simulink model "closedloopsystem"  (R2018a)
settings: Solver=VariableStepAuto  StartTime=0.0  StopTime=25  RelTol=1e-3
values from neighbouring files (symbols this model uses):
  b = 0.1    [DC_Motormfile.m]
  JM = 0.4    [DC_Motormfile.m]
  KE = 0.12    [DC_Motormfile.m]    (also in pid.m)
  KT = 0.25    [DC_Motormfile.m]    (also in pid.m)
  L = 493*10^-9    (= 4.93e-07)    [DC_Motormfile.m]    (also in pid.m)
  R = 5.3*10^-3    (= 0.0053)    [DC_Motormfile.m]    (also in pid.m)
  Scaling_Velocity = Sc/(Cw)*Rg*KE    (= 4.865)    [pid.m]
libraries: simulink x1
settings Model: Creator=MAFAZ  LastModifiedBy=MAFAZ

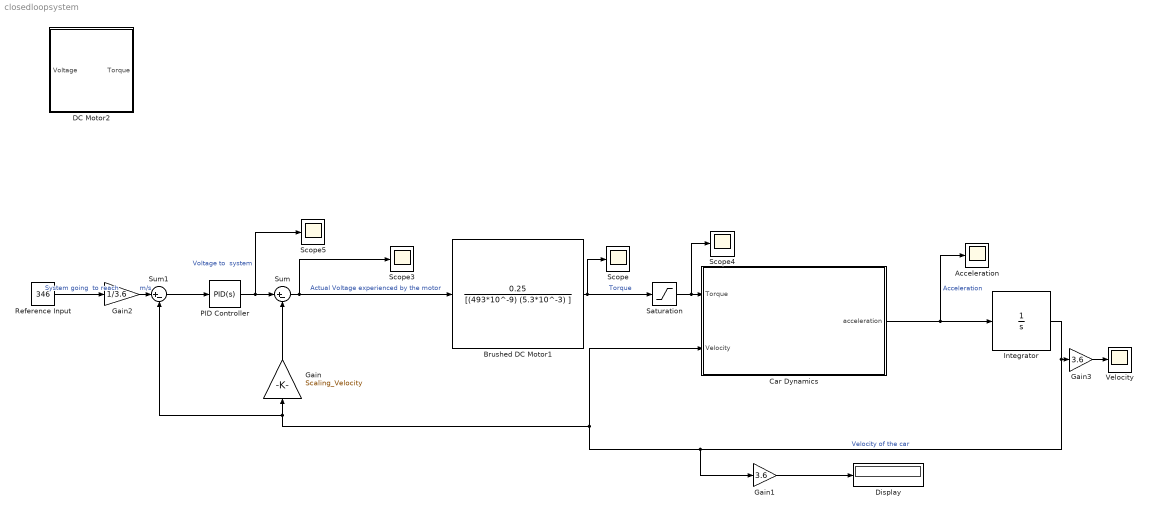
== system closedloopsystem ==
  Acceleration : Scope
  Brushed DC Motor1 : TransferFcn  Numerator=[0.25]  Denominator=[(493*10^-9) (5.3*10^-3) ]
  Car Dynamics : MATLAB Function  TreatAsAtomicUnit=on
  DC Motor2 : Subsystem
  Display : Display
  Gain : Gain  Gain=Scaling_Velocity
  Gain1 : Gain  Gain=3.6
  Gain2 : Gain  Gain=1/3.6
  Gain3 : Gain  Gain=3.6
  Integrator : Integrator
  PID Controller : simulink/Continuous/PID Controller  Controller=PID  TimeDomain=Continuous-time  SampleTime=-1  IntegratorMethod=Forward Euler  FilterMethod=Forward Euler  Form=Parallel  UseFilter=on  ControllerParametersSource=internal  P=1000000  I=0  D=0  N=100  InitialConditionSource=internal  InitialConditionForIntegrator=0  InitialConditionForFilter=0  ExternalReset=none  LimitOutput=on  UpperSaturationLimit=346  LowerSaturationLimit=0  LinearizeAsGain=on  AntiWindupMode=none  Kb=1  TrackingMode=off  Kt=1  PParamMin=[]  PParamMax=[]  IParamMin=[]  IParamMax=[]  DParamMin=[]  DParamMax=[]  NParamMin=[]  NParamMax=[]  KbParamMin=[]  KbParamMax=[]  KtParamMin=[]  KtParamMax=[]  POutMin=[]  POutMax=[]  IOutMin=[]  IOutMax=[]  DOutMin=[]  DOutMax=[]  NOutMin=[]  NOutMax=[]  KbOutMin=[]  KbOutMax=[]  KtOutMin=[]  KtOutMax=[]  IntegratorOutMin=[]  IntegratorOutMax=[]  FilterOutMin=[]  FilterOutMax=[]  SumOutMin=[]  SumOutMax=[]  SumI1OutMin=[]  SumI1OutMax=[]  SumI2OutMin=[]  SumI2OutMax=[]  SumI3OutMin=[]  SumI3OutMax=[]  SumDOutMin=[]  SumDOutMax=[]  SaturationOutMin=[]  SaturationOutMax=[]  IntegratorContinuousStateAttributes=''  IntegratorStateMustResolveToSignalObject=off  IntegratorRTWStateStorageClass=Auto  FilterContinuousStateAttributes=''  FilterStateMustResolveToSignalObject=off  FilterRTWStateStorageClass=Auto  DifferentiatorICPrevScaledInput=0  DifferentiatorOutMin=[]  DifferentiatorOutMax=[]  FilterDiffOutCoefMin=[]  FilterDiffOutCoefMax=[]  SumDenOutMin=[]  SumDenOutMax=[]  SumNumOutMin=[]  SumNumOutMax=[]  ReciprocalOutMin=[]  ReciprocalOutMax=[]  DivideOutMin=[]  DivideOutMax=[]  TunerSelectOption=Transfer Function Based (PID Tuner App)
  Reference Input : Constant  Value=346
  Saturation : Saturate  UpperLimit=600  LowerLimit=0
  Scope{,3..5} (4 alike) : Scope
  Sum : Sum  Inputs=|+-
  Sum1 : Sum  Inputs=|+-
  Velocity : Scope
  wires:
  PID Controller/1 -> Scope5/1, Sum/1  "Voltage to  system"
  Gain/1 -> Sum/2
  Brushed DC Motor1/1 -> Scope/1, Saturation/1  "Torque"
  Car Dynamics/1(acceleration) -> Acceleration/1, Integrator/1  "Acceleration"
  Integrator/1 -> Gain3/1, Gain1/1, Sum1/2, Gain/1, Car Dynamics/2(Velocity)  "Velocity of the car"
  Sum/1 -> Brushed DC Motor1/1, Scope3/1  "Actual Voltage experienced by the motor"
  Gain1/1 -> Display/1
  Saturation/1 -> Scope4/1, Car Dynamics/1(Torque)
  Reference Input/1 -> Gain2/1  "System going  to reach"
  Gain2/1 -> Sum1/1  "m/s"
  Sum1/1 -> PID Controller/1
  Gain3/1 -> Velocity/1

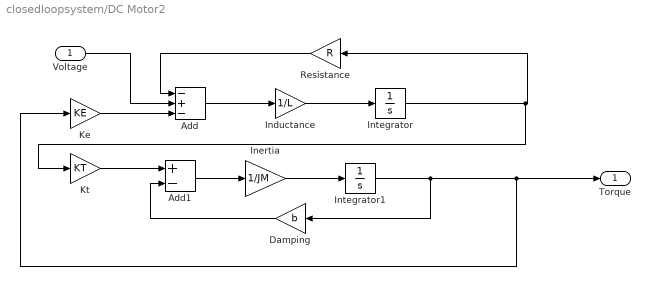
== system closedloopsystem/DC Motor2 ==
  Voltage : Inport
  Add : Sum  Inputs=-+-
  Add1 : Sum  Inputs=+-
  Damping : Gain  Gain=b
  Inductance : Gain  Gain=1/L
  Inertia : Gain  Gain=1/JM
  Integrator : Integrator
  Integrator1 : Integrator
  Ke : Gain  Gain=KE
  Kt : Gain  Gain=KT
  Resistance : Gain  Gain=R
  Torque : Outport
  wires:
  Damping/1 -> Add1/2
  Add1/1 -> Inertia/1
  Integrator/1 -> Kt/1, Resistance/1
  Inertia/1 -> Integrator1/1
  Ke/1 -> Add/3
  Add/1 -> Inductance/1
  Voltage/1 -> Add/2
  Inductance/1 -> Integrator/1
  Integrator1/1 -> Damping/1, Torque/1, Ke/1
  Kt/1 -> Add1/1
  Resistance/1 -> Add/1

== matlab function closedloopsystem/Car Dynamics ==
  data: Torque input; acceleration output; Velocity input
function acceleration = fcn(Torque, Velocity)
acceleration = (40.5*Torque*0.6-413-0.3381*Velocity^2)/2108;
